simulink model "chirp_excite"  (R2012b)
settings: Solver=FixedStepDiscrete  StartTime=0.0  StopTime=Tfinal  RelTol=1e-3
values from neighbouring files (symbols this model uses):
  AMP1 = 10    [runtests.m]    (also in runtests_lookuptable.m = 100*kamp.^T.*cos(PHASE_1+(2*pi*f0.*(k.^T-1)/log(k)) ))
  AMP2 = 10    [runtests.m]    (also in runtests_lookuptable.m = 100*kamp.^T.*cos(PHASE_2+(2*pi*f0.*(k.^T-1)/log(k)) ))
  Tfinal = 240    [runtests.m]    (also in runtests_lookuptable.m)
  Ts = 0.001    [runtests.m]    (also in runtests_lookuptable.m)
undefined symbols (not defined in the file or in its folder): National_Instruments, PCI
libraries: rtwinlib x2, dspsrcs4 x2, simulink x1
settings Model: SimulationMode=external  ExtModeTrigDuration=1400000  ExtModeArchiveMode=auto  ExtModeArchiveFileName=dataarch  ExtModeArchiveDirName=.\  Creator=f.cardoso-ribeiro  LastModifiedBy=f.cardoso-ribeiro
settings SolverCC: AutoInsertRateTranBlk=on
settings DataIOCC: LimitDataPoints=off  SaveOutput=off  SignalLogging=off  DSMLogging=off  SaveTime=off
settings HardwareCC: ProdIntDivRoundTo=Zero  ProdEndianess=LittleEndian  ProdHWDeviceType=Generic->32-bit x86 compatible
settings RTWCC: SystemTargetFile=rtwin.tlc  TemplateMakefile=rtwin.tmf  Description=Real-Time Windows Target  RTWVerbose=off  ProcessScript=rtwin_make_rtw_hook  RTWCompilerOptimization=On
settings CodeAppCC: MaxIdLength=95
settings RTWinTargetCC: TargetLibSuffix=_rtwin.lib  TargetPreCompLibLocation=C:\Program Files\MATLAB\R2012b\toolbox\rtw\targets\rtwin\lib\win64  CodeReplacementLibrary=ANSI_C  RTWinDir=C:/PROGRA~1/MATLAB/R2012b/toolbox/rtw/targets/rtwin  TargetArch=win64

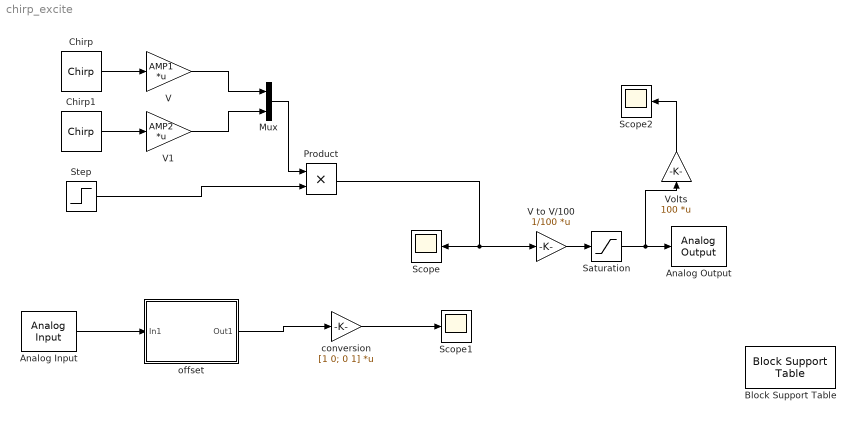
== system chirp_excite ==
  Analog Input : rtwinlib/Analog Input  SampleTime=Ts  MaxMissedTicks=10  ShowMissedTicks=off  YieldWhenWaiting=off  DrvName=National_Instruments/PCI-6024E  DrvAddress=4294967295  DrvOptions=[1 0 0 0 0 0]  Channels=[1 2]  RangeMode=1  VoltRange=1  DataType=1
      settings: AttributesFormatString=National Instruments\nPCI-6024E [auto]
  Analog Output : rtwinlib/Analog Output  SampleTime=Ts  MaxMissedTicks=10  ShowMissedTicks=off  YieldWhenWaiting=off  DrvName=National_Instruments/PCI-6024E  DrvAddress=4294967295  DrvOptions=[1 0 0 0 0 0]  Channels=[1 2]  RangeMode=1  VoltRange=1  InitialValue=0  FinalValue=0
      settings: AttributesFormatString=National Instruments\nPCI-6024E [auto]
  Block Support Table : simulink/Model-Wide Utilities/Block Support Table
  Chirp : dspsrcs4/Chirp  sweep=Logarithmic  mode=Bidirectional  f0=0.2  f1=200  t1=Tfinal-20  Tsweep=Tfinal-20  phase=PHASE_1  Ts=Ts  spf=1  datatype=Double
  Chirp1 : dspsrcs4/Chirp  sweep=Logarithmic  mode=Bidirectional  f0=0.2  f1=200  t1=Tfinal-20  Tsweep=Tfinal-20  phase=PHASE_2  Ts=Ts  spf=1  datatype=Double
  Mux : Mux  Inputs=2
  Product : Product  RndMeth=Zero
  Saturation : Saturate  UpperLimit=1.5  LowerLimit=-1.5
  Scope : Scope
      settings: YMin=-50  YMax=50  SaveName=input
  Scope1 : Scope
      settings: TimeRange=120  YMin=-0.045  YMax=0.035  SaveName=output
  Scope2 : Scope
      settings: YMin=-10  YMax=10  SaveName=input1
  Step : Step  Time=Tfinal-20  Before=1  After=0  SampleTime=0
  V : Gain  Gain=AMP1  Multiplication=Matrix(K*u)
  "V to V/100 " : Gain  Gain=1/100  Multiplication=Matrix(K*u)
  V1 : Gain  Gain=AMP2  Multiplication=Matrix(K*u)
  Volts : Gain  Gain=100  Multiplication=Matrix(K*u)
  conversion : Gain  Gain=[1 0; 0 1]  Multiplication=Matrix(K*u)
  offset : Subsystem
  wires:
  Saturation/1 -> Volts/1, Analog Output/1
  Product/1 -> "V to V/100 "/1, Scope/1
  "V to V/100 "/1 -> Saturation/1
  Step/1 -> Product/2
  Chirp/1 -> V/1
  V/1 -> Mux/1
  conversion/1 -> Scope1/1
  Analog Input/1 -> offset/1(In1)
  offset/1(Out1) -> conversion/1
  Chirp1/1 -> V1/1
  V1/1 -> Mux/2
  Mux/1 -> Product/1
  Volts/1 -> Scope2/1

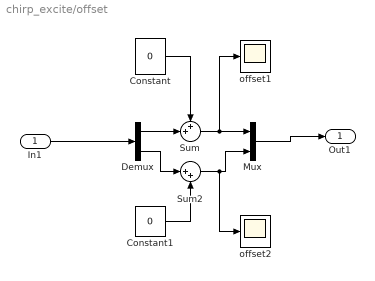
== system chirp_excite/offset ==
  In1 : Inport
  Constant : Constant  Value=0
  Constant1 : Constant  Value=0
  Demux : Demux  Outputs=2
  Mux : Mux  Inputs=2
  Sum : Sum  Inputs=++|
  Sum2 : Sum  Inputs=|++
  offset1 : Scope
      settings: YMin=-1.5  YMax=1.5  SaveName=output2
  offset2 : Scope
      settings: TimeRange=1200  YMin=-0.018  YMax=0.003  SaveName=output1
  Out1 : Outport
  wires:
  In1/1 -> Demux/1
  Mux/1 -> Out1/1
  Constant1/1 -> Sum2/2
  Constant/1 -> Sum/1
  Demux/2 -> Sum2/1
  Sum2/1 -> offset2/1, Mux/2
  Sum/1 -> offset1/1, Mux/1
  Demux/1 -> Sum/2
